simulink model "ec_generic_block"  (Simulink 7.0)
settings: Solver=FixedStepDiscrete  StartTime=0.0  StopTime=tend  FixedStep=ts  RelTol=1e-3
model workspace: external: M-Code (data not in the file)
Description:
  | Model for a generic ethercat stack
settings Model: Creator=root  LastModifiedBy=root  SimulationMode=external  ExtModeAutoUpdateStatusClock=off
settings DebuggingCC: SaveWithParameterizedLinksMsg=none  SignalResolutionControl=TryResolveAllWithWarning  MultiTaskDSMMsg=warning  MultiTaskCondExecSysMsg=none  StrictBusMsg=None
settings RTWCC: SystemTargetFile=ectarget.tlc  MakeCommand="make_rtw OPTS=\"-DNETIF_ID=0 -DEC_GENERIC\""  TemplateMakefile=ec_unix.tmf  Description=Ethercattarget Real-Time Target for PREEMPT-RT/Linux  ProcessScript=ectarget_make_rtw_hook  IncludeERTFirstTime=on
settings GRTTargetCC: TargetFcnLib=ansi_tfl_tmw.mat  ExtMode=on

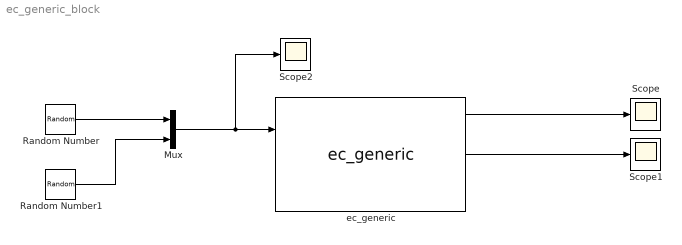
== system ec_generic_block ==
  Mux : Mux  Inputs=2
  Random Number : RandomNumber  Variance=3  SampleTime=0
  Random Number1 : RandomNumber  Variance=3  Seed=122345  SampleTime=0
  Scope : Scope
      settings: TimeRange=1  YMin=-2  YMax=2.5  SaveName=adc  DataFormat=Array
  Scope1 : Scope
      settings: TimeRange=1  YMin=-10000  YMax=20000
  Scope2 : Scope
      settings: TimeRange=1  YMin=-2  YMax=2.5  SaveName=dac  DataFormat=Array
  ec_generic : S-Function  FunctionName=ec_generic
      mask init:
      | ports
      mask Display:
      | port_label('output',1,['ADC [',num2str(NADC),']'])
      | port_label('output',2,['ENC [',num2str(NENC),']'])
      | port_label('output',3,['DI [',num2str(NDIN),']'])
      | port_label('input',1,['DAC [',num2str(NDAC),']'])
      | port_label('input',2,['DO [',num2str(NDOUT),']'])
  wires:
  ec_generic/1 -> Scope/1
  ec_generic/2 -> Scope1/1
  Mux/1 -> ec_generic/1, Scope2/1
  Random Number/1 -> Mux/1
  Random Number1/1 -> Mux/2
